simulink model "flow_control_for"  (R2013b)
settings: Solver=ode45  StartTime=0.0  StopTime=10  RelTol=1e-3
settings Model: Creator=Administrator  LastModifiedBy=Administrator

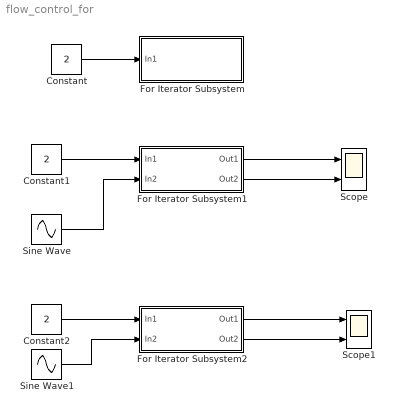
== system flow_control_for ==
  Constant : Constant  Value=2
  Constant1 : Constant  Value=2
  Constant2 : Constant  Value=2
  For Iterator Subsystem : Subsystem  TreatAsAtomicUnit=on
  For Iterator Subsystem1 : Subsystem  TreatAsAtomicUnit=on
  For Iterator Subsystem2 : Subsystem  TreatAsAtomicUnit=on
  Scope : Scope  NumInputPorts=2
      settings: YMin=-5~-5  YMax=5~5
  Scope1 : Scope  NumInputPorts=2
      settings: YMin=-5~-5  YMax=5~5  SaveName=ScopeData2
  Sine Wave : Sin  Amplitude=11  SampleTime=0
  Sine Wave1 : Sin  Amplitude=11  SampleTime=0
  wires:
  Constant/1 -> For Iterator Subsystem/1(In1)
  Constant1/1 -> For Iterator Subsystem1/1(In1)
  For Iterator Subsystem1/1(Out1) -> Scope/1
  For Iterator Subsystem1/2(Out2) -> Scope/2
  Sine Wave/1 -> For Iterator Subsystem1/2(In2)
  Constant2/1 -> For Iterator Subsystem2/1(In1)
  For Iterator Subsystem2/1(Out1) -> Scope1/1
  For Iterator Subsystem2/2(Out2) -> Scope1/2
  Sine Wave1/1 -> For Iterator Subsystem2/2(In2)

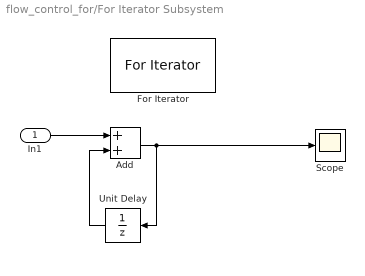
== system flow_control_for/For Iterator Subsystem ==
  In1 : Inport
  Add : Sum
  For Iterator : ForIterator  ShowIterationPort=off
  Scope : Scope
      settings: YMin=-1  YMax=100
  Unit Delay : UnitDelay  SampleTime=-1
  wires:
  In1/1 -> Add/1
  Add/1 -> Scope/1, Unit Delay/1
  Unit Delay/1 -> Add/2

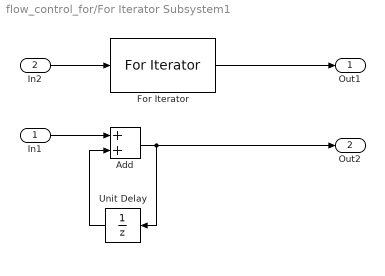
== system flow_control_for/For Iterator Subsystem1 ==
  In1 : Inport
  In2 : Inport  Port=2
  Add : Sum
  For Iterator : ForIterator  IterationSource=external  IterationVariableDataType=double
  Unit Delay : UnitDelay  SampleTime=-1
  Out1 : Outport
  Out2 : Outport  Port=2
  wires:
  In1/1 -> Add/1
  Add/1 -> Out2/1, Unit Delay/1
  Unit Delay/1 -> Add/2
  For Iterator/1 -> Out1/1
  In2/1 -> For Iterator/1

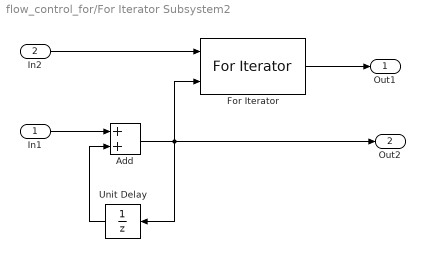
== system flow_control_for/For Iterator Subsystem2 ==
  In1 : Inport
  In2 : Inport  Port=2
  Add : Sum
  For Iterator : ForIterator  IterationSource=external  ExternalIncrement=on  IterationVariableDataType=double
  Unit Delay : UnitDelay  SampleTime=-1
  Out1 : Outport
  Out2 : Outport  Port=2
  wires:
  Unit Delay/1 -> Add/2
  For Iterator/1 -> Out1/1
  In2/1 -> For Iterator/1
  Add/1 -> For Iterator/2, Out2/1, Unit Delay/1
  In1/1 -> Add/1
